simulink model "Simulate_CycleGAN"  (Simulink 10.2)
settings: Solver=ode45  StartTime=0.0  StopTime=30  RelTol=1e-3  EnableMultiTasking=on
libraries: slpidlib x4
settings Model: Creator=Administrator  LastModifiedBy=hunter
settings SolverCC: ZeroCrossControl=DisableAll
settings DataIOCC: LimitDataPoints=on
settings OptimizationCC: ExpressionDepthLimit=2147483647
settings DebuggingCC: SolverPrmCheckMsg=warning  StateNameClashWarn=warning

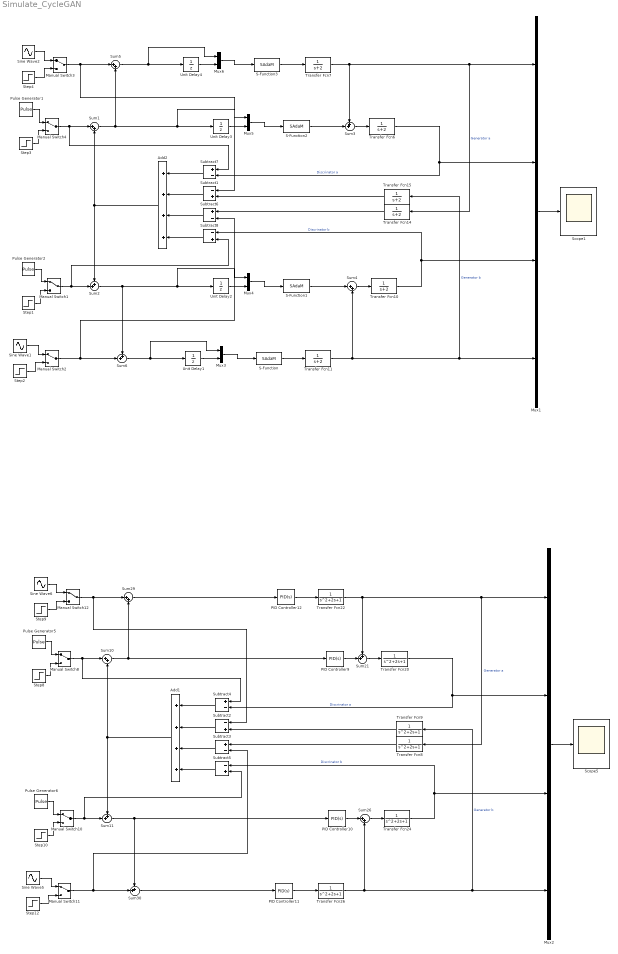
== system Simulate_CycleGAN ==
  Add1 : Sum  Inputs=++++
  Add2 : Sum  Inputs=++++
  Manual Switch{1..4,8,10..12} (8 alike) : ManualSwitch
  Mux1 : Mux
  Mux2 : Mux
  Mux{3..6} (4 alike) : Mux  Inputs=2
  PID Controller{9..12} (4 alike) : slpidlib/PID Controller  Controller=PID  Form=Parallel  TimeDomain=Continuous-time  UseExternalTs=off  SampleTime=-1  IntegratorMethod=Forward Euler  FilterMethod=Forward Euler  ControllerParametersSource=internal  P=1  I=5  D=100  UseFilter=on  N=100  TunerSelectOption=Transfer Function Based (PID Tuner App)  InitialConditionSource=internal  InitialConditionForIntegrator=0  InitialConditionForFilter=0  DifferentiatorICPrevScaledInput=0  ExternalReset=none  TrackingMode=off  Kt=1  LimitOutput=off  SatLimitsSource=internal  UpperSaturationLimit=inf  LowerSaturationLimit=-inf  LinearizeAsGain=on  AntiWindupMode=none  Kb=1  POutMin=[]  POutMax=[]  IOutMin=[]  IOutMax=[]  DOutMin=[]  DOutMax=[]  NOutMin=[]  NOutMax=[]  SumOutMin=[]  SumOutMax=[]  SaturationOutMin=[]  SaturationOutMax=[]  PParamMin=[]  PParamMax=[]  IParamMin=[]  IParamMax=[]  DParamMin=[]  DParamMax=[]  NParamMin=[]  NParamMax=[]  KbParamMin=[]  KbParamMax=[]  KtParamMin=[]  KtParamMax=[]  KbOutMin=[]  KbOutMax=[]  KtOutMin=[]  KtOutMax=[]  IntegratorOutMin=[]  IntegratorOutMax=[]  FilterOutMin=[]  FilterOutMax=[]  SumI1OutMin=[]  SumI1OutMax=[]  SumI2OutMin=[]  SumI2OutMax=[]  SumI3OutMin=[]  SumI3OutMax=[]  SumI4OutMin=[]  SumI4OutMax=[]  SumDOutMin=[]  SumDOutMax=[]  DifferentiatorOutMin=[]  DifferentiatorOutMax=[]  FilterDiffOutCoefMin=[]  FilterDiffOutCoefMax=[]  ReciprocalOutMin=[]  ReciprocalOutMax=[]  SumDenOutMin=[]  SumDenOutMax=[]  SumNumOutMin=[]  SumNumOutMax=[]  DivideOutMin=[]  DivideOutMax=[]  UdiffTsProdOutMin=[]  UdiffTsProdOutMax=[]  NTsProdOutMin=[]  NTsProdOutMax=[]  UintegralTsProdOutMin=[]  UintegralTsProdOutMax=[]  UngainTsProdOutMin=[]  UngainTsProdOutMax=[]  IntegratorContinuousStateAttributes=''  IntegratorStateMustResolveToSignalObject=off  IntegratorRTWStateStorageClass=Auto  FilterContinuousStateAttributes=''  FilterStateMustResolveToSignalObject=off  FilterRTWStateStorageClass=Auto  ParallelPVariant=InternalParameters  IdealPVariant=Disabled  IVariant=InternalParameters  DVariant=InternalParameters  IntegratorVariant=Continuous  SatVariant=Disabled  AWVariant=Passthrough  PCopyVariant=Disabled  TRVariant=Disabled  FdbkBlocksVariant=Forward  IdealPFdbkVariant=Disabled  SatFdbkVariant=Disabled  DerivativeFilterVariant=ContFilter  NVariant=InternalParameters  NCopyVariant=Disabled  FilterICVariant=InternalICsFilter  IntegratorICVariant=InternalICs  ExternalResetVariant=Disabled  TRSumVariant=Passthrough  SumFdbkVariant=Disabled  SumVariant=Sum_PID  TsampFilterVariant=InternalTs  TsampNgainVariant=Passthrough  TsampIntegralVariant=Passthrough  ExternalSaturationOutDataTypeStr=Inherit: Same as second input
  Pulse Generator{1..2,5..6} (4 alike) : DiscretePulseGenerator  PulseType=Time based  Period=10  PulseWidth=50
  S-Function{,1..3} (4 alike) : S-Function  FunctionName=SAdaM  SFunctionDeploymentMode=off  EnableBusSupport=off
  Scope1 : Scope
  Scope5 : Scope
  Sine Wave1 : Sin  Frequency=pi*0.2  Phase=pi  SampleTime=0
  Sine Wave2 : Sin  Frequency=pi*0.2  SampleTime=0
  Sine Wave5 : Sin  Frequency=pi*0.2  Phase=pi  SampleTime=0
  Sine Wave6 : Sin  Frequency=pi*0.2  SampleTime=0
  Step{1..3,8,10,12} (6 alike) : Step  Time=0  SampleTime=0
  Step4 : Step  Time=0  After=-1  SampleTime=0
  Step9 : Step  Time=0  After=-1  SampleTime=0
  Subtract{1..2,5,8} (4 alike) : Sum  Inputs=-+
  Subtract{3..4,6..7} (4 alike) : Sum  Inputs=+-
  Sum{1,4..5,10,26,29} (6 alike) : Sum  Inputs=|++
  Sum{2..3,6,11,21,30} (6 alike) : Sum  Inputs=++|
  Transfer Fcn{6..7,10..11,14..15} (6 alike) : TransferFcn  Denominator=[1 2]
  Transfer Fcn{8..9,20,22,24,26} (6 alike) : TransferFcn
  Unit Delay{1..4} (4 alike) : UnitDelay  SampleTime=-1  HasFrameUpgradeWarning=on
  wires:
  Add1/1 -> Sum11/1, Sum10/2
  Transfer Fcn26/1 -> Transfer Fcn9/1, Mux2/4, Sum26/2  "Generator b"
  Step12/1 -> Manual Switch11/2
  Transfer Fcn22/1 -> Sum21/1, Transfer Fcn8/1, Mux2/1  "Generator a"
  Pulse Generator6/1 -> Manual Switch10/1
  Step10/1 -> Manual Switch10/2
  Manual Switch12/1 -> Subtract2/1, Sum29/1
  Sine Wave6/1 -> Manual Switch12/1
  Transfer Fcn20/1 -> Subtract4/2, Mux2/2  "Discrinator a"
  Sum21/1 -> Transfer Fcn20/1
  Step9/1 -> Manual Switch12/2
  Step8/1 -> Manual Switch8/2
  PID Controller12/1 -> Transfer Fcn22/1
  Subtract5/1 -> Add1/4
  PID Controller10/1 -> Sum26/1
  Transfer Fcn24/1 -> Subtract5/1, Mux2/3  "Discrinator b"
  PID Controller9/1 -> Sum21/2
  Subtract3/1 -> Add1/3
  Manual Switch8/1 -> Subtract4/1, Sum10/1
  Pulse Generator5/1 -> Manual Switch8/1
  Mux2/1 -> Scope5/1
  Subtract2/1 -> Add1/2
  Transfer Fcn8/1 -> Subtract3/1
  Sum26/1 -> Transfer Fcn24/1
  PID Controller11/1 -> Transfer Fcn26/1
  Sine Wave5/1 -> Manual Switch11/1
  Subtract4/1 -> Add1/1
  Manual Switch11/1 -> Subtract3/2, Sum30/2
  Transfer Fcn9/1 -> Subtract2/2
  Manual Switch10/1 -> Subtract5/2, Sum11/2
  Manual Switch2/1 -> Subtract6/2, Sum6/2
  S-Function1/1 -> Sum4/1
  Transfer Fcn7/1 -> Sum3/1, Transfer Fcn14/1, Mux1/1  "Generator a"
  Step3/1 -> Manual Switch4/2
  Sine Wave2/1 -> Manual Switch3/1
  Transfer Fcn6/1 -> Subtract7/2, Mux1/2  "Discrinator a"
  S-Function3/1 -> Transfer Fcn7/1
  Subtract7/1 -> Add2/1
  Transfer Fcn14/1 -> Subtract6/1
  S-Function/1 -> Transfer Fcn11/1
  Pulse Generator2/1 -> Manual Switch1/1
  Subtract8/1 -> Add2/4
  Manual Switch4/1 -> Subtract7/1, Sum1/1
  Step4/1 -> Manual Switch3/2
  Sum3/1 -> Transfer Fcn6/1
  Add2/1 -> Sum2/1, Sum1/2
  Transfer Fcn11/1 -> Transfer Fcn15/1, Mux1/4, Sum4/2  "Generator b"
  Transfer Fcn15/1 -> Subtract1/2
  Pulse Generator1/1 -> Manual Switch4/1
  Sum4/1 -> Transfer Fcn10/1
  Sine Wave1/1 -> Manual Switch2/1
  Step1/1 -> Manual Switch1/2
  Manual Switch3/1 -> Subtract1/1, Sum5/1
  S-Function2/1 -> Sum3/2
  Mux1/1 -> Scope1/1
  Transfer Fcn10/1 -> Subtract8/1, Mux1/3  "Discrinator b"
  Subtract1/1 -> Add2/2
  Manual Switch1/1 -> Subtract8/2, Sum2/2
  Step2/1 -> Manual Switch2/2
  Subtract6/1 -> Add2/3
  Sum6/1 -> Unit Delay1/1, Mux3/1
  Unit Delay1/1 -> Mux3/2
  Mux3/1 -> S-Function/1
  Mux4/1 -> S-Function1/1
  Unit Delay2/1 -> Mux4/2
  Sum2/1 -> Unit Delay2/1, Mux4/1, Sum6/1
  Mux5/1 -> S-Function2/1
  Unit Delay3/1 -> Mux5/2
  Sum1/1 -> Unit Delay3/1, Mux5/1, Sum5/2
  Mux6/1 -> S-Function3/1
  Unit Delay4/1 -> Mux6/2
  Sum5/1 -> Unit Delay4/1, Mux6/1
  Sum29/1 -> PID Controller12/1
  Sum10/1 -> PID Controller9/1, Sum29/2
  Sum11/1 -> PID Controller10/1, Sum30/1
  Sum30/1 -> PID Controller11/1
